simulink model "hl20airframe"  (Simulink 4.00)
settings: Solver=ode45  StartTime=0.0  StopTime=1000.0  RelTol=1e-3
PreLoadFcn:
  | init_hl20
values from neighbouring files (symbols this model uses):
  alpha_vec_Cn0 = [-10 -5 0 5 10 15 20 25 30]    [init_hl20.m]
  b_ref = 13.89/m2ft    (= 4.23367186452)    [init_hl20.m]
  beta_vec_Cn0 = [0 2 5 10]    [init_hl20.m]
  Clbeta = -0.00787    [init_hl20.m]
  Cm0 = reshape(temp(:,2),length(beta_vec_0),length(alpha_vec_0))    [init_hl20.m]
  CX0 = -reshape(temp(:,3),length(beta_vec_0),length(alpha_vec_0))    [init_hl20.m]
  CYbeta = -0.01242    [init_hl20.m]
  CZ0 = -reshape(temp(:,1),length(beta_vec_0),length(alpha_vec_0))    [init_hl20.m]
  d2r = pi/180    (= 0.0174532925199)    [init_hl20.m]
  d_ref = 28.24/m2ft    (= 8.60755172456)    [init_hl20.m]
  Inertia = diag([Ixx Iyy Izz])    [init_hl20.m]
  mass = massBody+massFuel    (= 11738.9844962)    [init_hl20.m]
  S_ref = 286.45/m2ft^2    (= 26.6120741048)    [init_hl20.m]
  x_cg = 0.575*len_veh    (= 4.78635044684)    [init_hl20.m]
  x_ref = 0.54*len_veh    (= 4.49500737616)    [init_hl20.m]
undefined symbols (not defined in the file or in its folder): Light
libraries: simulink3 x40, aerolibwind x3, aerolib6dof x1, aerolibatmos x1, aerolibgravity x1, aerolibtransform x1
settings Model: Creator=sgage  LastModifiedBy=sgage  OptimizeBlockIOStorage=off

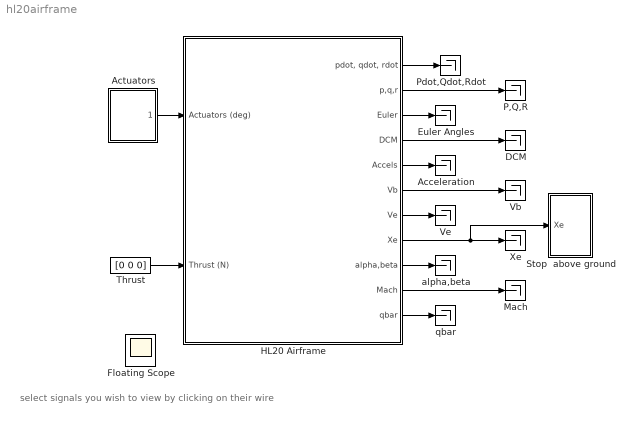
== system hl20airframe ==
  note: select signals you wish to view
      | by clicking on their wire
  Acceleration : Terminator
  Actuators : Subsystem
      settings: RTWFcnNameOpts=Auto  RTWFileNameOpts=Auto
  DCM : Terminator
  Euler Angles : Terminator
  Floating Scope : Scope
      settings: Floating=on  TimeRange=10  YMin=-7500  YMax=1000  SaveToWorkspace=off  SaveName=ScopeData  LimitDataPoints=on  MaxDataPoints=5000
  HL20 Airframe : Subsystem
      settings: RTWFcnNameOpts=Auto  RTWFileNameOpts=Auto
      mask Display: image(imread('aeroblk_HL20pic.jpg','jpg'))
  Mach : Terminator
  P,Q,R : Terminator
  Pdot,Qdot,Rdot : Terminator
  Stop  above ground : Subsystem
      settings: RTWFcnNameOpts=Auto  RTWFileNameOpts=Auto
  Thrust : Constant  Value=[0 0 0]
  Vb : Terminator
  Ve : Terminator
  Xe : Terminator
  alpha,beta : Terminator
  qbar : Terminator
  wires:
  Thrust/1 -> HL20 Airframe/2(Thrust (N))
  Actuators/1(Positions) -> HL20 Airframe/1(Actuators (deg))
  HL20 Airframe/11(qbar) -> qbar/1
  HL20 Airframe/3(Euler) -> Euler Angles/1
  HL20 Airframe/5(Accels) -> Acceleration/1
  HL20 Airframe/6(Vb) -> Vb/1
  HL20 Airframe/1("pdot, qdot, rdot") -> Pdot,Qdot,Rdot/1
  HL20 Airframe/2(p,q,r) -> P,Q,R/1
  HL20 Airframe/7(Ve) -> Ve/1
  HL20 Airframe/8(Xe) -> Xe/1, Stop  above ground/1(Xe)
  HL20 Airframe/10(Mach) -> Mach/1
  HL20 Airframe/9(alpha,beta) -> alpha,beta/1
  HL20 Airframe/4(DCM) -> DCM/1

== system hl20airframe/Actuators ==
  Bus Creator1 : BusCreator  Inputs=6
  Constant : Constant  Value=0
  Sine Wave : Sin  SineType=Time-based  Amplitude=1  Bias=10  Frequency=1  Phase=0  Samples=10  SampleTime=0  Offset=0
  "aileron " : Saturate  UpperLimit=30  LowerLimit=-30  LinearizeAsGain=on
  elevator : Saturate  UpperLimit=30  LowerLimit=-30  LinearizeAsGain=on
  flap (diff) : Saturate  UpperLimit=60  LowerLimit=-60  LinearizeAsGain=on
  flap (neg) : Saturate  UpperLimit=0  LowerLimit=-60  LinearizeAsGain=on
  flap (pos) : Saturate  UpperLimit=60  LowerLimit=0  LinearizeAsGain=on
  rudder : Saturate  UpperLimit=60  LowerLimit=-60  LinearizeAsGain=on
  Positions : Outport  Port=1
  wires:
  Bus Creator1/1 -> Positions/1
  flap (diff)/1 -> Bus Creator1/6  "Flap(diff)"
  flap (neg)/1 -> Bus Creator1/5  "Flap(neg)"
  rudder/1 -> Bus Creator1/3  "Rudder"
  elevator/1 -> Bus Creator1/2  "Elevator"
  "aileron "/1 -> Bus Creator1/1  "Aileron"
  flap (pos)/1 -> Bus Creator1/4  "Flap(pos)"
  Constant/1 -> rudder/1, flap (diff)/1, flap (neg)/1, flap (pos)/1, "aileron "/1
  Sine Wave/1 -> elevator/1

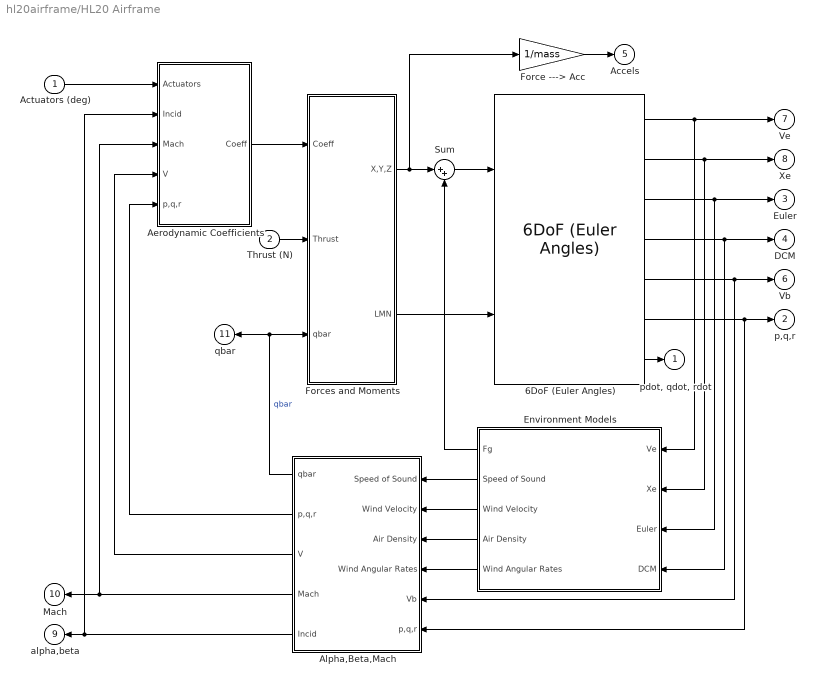
== system hl20airframe/HL20 Airframe ==
  Actuators (deg) : Inport  Port=1  LatchInput=off
  Thrust (N) : Inport  Port=2  LatchInput=off
  6DoF (Euler Angles) : aerolib6dof/6DoF (Euler Angles)  xme_0=xme_0  Vm_0=Vmw  eul_0=Euler_0  pm_0=pm_0  Mass=mass  Inertia=Inertia
  Aerodynamic Coefficients : Subsystem
      settings: RTWFcnNameOpts=Auto  RTWFileNameOpts=Auto
  Alpha,Beta,Mach : Subsystem  Orientation=left
      settings: RTWFcnNameOpts=Auto  RTWFileNameOpts=Auto
  Environment Models : Subsystem  Orientation=left
      settings: RTWFcnNameOpts=Auto  RTWFileNameOpts=Auto
  Force ---> Acc : Gain  Gain=1/mass  Multiplication=Element-wise(K.*u)  SaturateOnIntegerOverflow=on
  Forces and Moments : Subsystem
      settings: RTWFcnNameOpts=Auto  RTWFileNameOpts=Auto
  Sum : Sum  Inputs=|++  SaturateOnIntegerOverflow=on
  "pdot, qdot, rdot" : Outport  Port=1  InitialOutput=0
  p,q,r : Outport  Port=2  InitialOutput=0
  Euler : Outport  Port=3  InitialOutput=0
  DCM : Outport  Port=4  InitialOutput=0
  Accels : Outport  Port=5  InitialOutput=0
  Vb : Outport  Port=6  InitialOutput=0
  Ve : Outport  Port=7  InitialOutput=0
  Xe : Outport  Port=8  InitialOutput=0
  alpha,beta : Outport  Orientation=left  Port=9  InitialOutput=0
  Mach : Outport  Orientation=left  Port=10  InitialOutput=0
  qbar : Outport  Orientation=left  Port=11  InitialOutput=0
  wires:
  6DoF (Euler Angles)/1 -> Environment Models/1(Ve), Ve/1
  6DoF (Euler Angles)/2 -> Environment Models/2(Xe), Xe/1
  6DoF (Euler Angles)/6 -> p,q,r/1, Alpha,Beta,Mach/6(p,q,r)
  Thrust (N)/1 -> Forces and Moments/2(Thrust)
  6DoF (Euler Angles)/7 -> "pdot, qdot, rdot"/1
  6DoF (Euler Angles)/4 -> DCM/1, Environment Models/4(DCM)
  6DoF (Euler Angles)/3 -> Environment Models/3(Euler), Euler/1
  Alpha,Beta,Mach/5(Incid) -> alpha,beta/1, Aerodynamic Coefficients/2(Incid)
  Aerodynamic Coefficients/1(Coeff) -> Forces and Moments/1(Coeff)
  Environment Models/3(Wind Velocity) -> Alpha,Beta,Mach/2(Wind Velocity)
  6DoF (Euler Angles)/5 -> Alpha,Beta,Mach/5(Vb), Vb/1
  Environment Models/2(Speed of Sound) -> Alpha,Beta,Mach/1(Speed of Sound)
  Environment Models/4(Air Density) -> Alpha,Beta,Mach/3(Air Density)
  Forces and Moments/2(LMN) -> 6DoF (Euler Angles)/2
  Alpha,Beta,Mach/1(qbar) -> Forces and Moments/3(qbar), qbar/1  "qbar"
  Forces and Moments/1(X,Y,Z) -> Sum/1, Force ---> Acc/1
  Sum/1 -> 6DoF (Euler Angles)/1
  Environment Models/1(Fg) -> Sum/2
  Force ---> Acc/1 -> Accels/1
  Actuators (deg)/1 -> Aerodynamic Coefficients/1(Actuators)
  Alpha,Beta,Mach/3(V) -> Aerodynamic Coefficients/4(V)
  Alpha,Beta,Mach/4(Mach) -> Aerodynamic Coefficients/3(Mach), Mach/1
  Alpha,Beta,Mach/2("p,q,r ") -> Aerodynamic Coefficients/5(p,q,r)
  Environment Models/5(Wind Angular Rates) -> Alpha,Beta,Mach/4(Wind Angular Rates)

== system hl20airframe/Stop  above ground ==
  Xe : Inport  Port=1  LatchInput=off
  1 meter from ground : Fcn  Expr=u[1] <= 2
  Abs : Abs  SaturateOnIntegerOverflow=on
  Selector : Selector  InputType=Vector  ElementSrc=Internal  Elements=3  RowSrc=Internal  Rows=1  ColumnSrc=Internal  Columns=1  InputPortWidth=3
  Stop Simulation : Stop
  wires:
  Selector/1 -> Abs/1
  1 meter from ground/1 -> Stop Simulation/1
  Xe/1 -> Selector/1
  Abs/1 -> 1 meter from ground/1

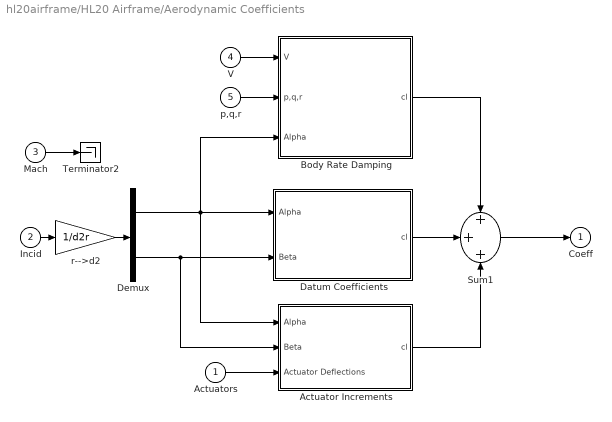
== system hl20airframe/HL20 Airframe/Aerodynamic Coefficients ==
  Actuators : Inport  Port=1  LatchInput=off
  Incid : Inport  Port=2  LatchInput=off
  Mach : Inport  Port=3  LatchInput=off
  V : Inport  Port=4  LatchInput=off
  p,q,r : Inport  Port=5  LatchInput=off
  Actuator Increments : Subsystem
      settings: RTWFcnNameOpts=Auto  RTWFileNameOpts=Auto
  Body Rate Damping : Subsystem
      settings: RTWFcnNameOpts=Auto  RTWFileNameOpts=Auto
  Datum Coefficients : Subsystem
      settings: RTWFcnNameOpts=Auto  RTWFileNameOpts=Auto
  Demux : Demux  Outputs=2  BusSelectionMode=off
  Sum1 : Sum  Inputs=+++  SaturateOnIntegerOverflow=on
  Terminator2 : Terminator
  r-->d2 : Gain  Gain=1/d2r  Multiplication=Element-wise(K.*u)  SaturateOnIntegerOverflow=on
  Coeff : Outport  Port=1  InitialOutput=0
  wires:
  Actuator Increments/1(cl) -> Sum1/3
  Body Rate Damping/1(cl) -> Sum1/1
  V/1 -> Body Rate Damping/1(V)
  Mach/1 -> Terminator2/1
  Demux/2 -> Actuator Increments/2(Beta), Datum Coefficients/2(Beta)
  Datum Coefficients/1(cl) -> Sum1/2
  Sum1/1 -> Coeff/1
  Actuators/1 -> Actuator Increments/3("Actuator Deflections ")
  r-->d2/1 -> Demux/1
  Incid/1 -> r-->d2/1
  p,q,r/1 -> Body Rate Damping/2(p,q,r)
  Demux/1 -> Actuator Increments/1(Alpha), Datum Coefficients/1(Alpha), Body Rate Damping/3(Alpha)

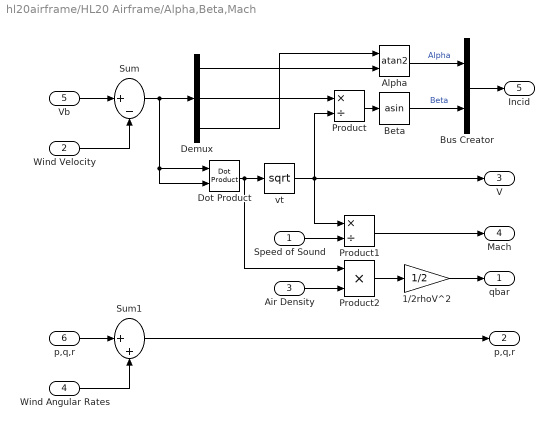
== system hl20airframe/HL20 Airframe/Alpha,Beta,Mach ==
  Speed of Sound : Inport  Port=1  LatchInput=off
  Wind Velocity : Inport  Port=2  LatchInput=off  PortDimensions=3
  Air Density : Inport  Port=3  LatchInput=off
  Wind Angular Rates : Inport  Port=4  LatchInput=off  PortDimensions=3
  Vb : Inport  Port=5  LatchInput=off  PortDimensions=3
  p,q,r : Inport  Port=6  LatchInput=off  PortDimensions=3
  1/2rhoV^2 : Gain  Gain=1/2  Multiplication=Element-wise(K.*u)  SaturateOnIntegerOverflow=on
  Alpha : Trigonometry  Operator=atan2  OutputSignalType=auto
  Beta : Trigonometry  Operator=asin  OutputSignalType=auto
  Bus Creator : BusCreator  Inputs=2
  Demux : Demux  Outputs=3  BusSelectionMode=off
  Dot Product : simulink3/Math/Dot Product
  Product : Product  Inputs=*/  Multiplication=Element-wise(.*)  SaturateOnIntegerOverflow=on
  Product1 : Product  Inputs=*/  Multiplication=Element-wise(.*)  SaturateOnIntegerOverflow=on
  Product2 : Product  Inputs=2  Multiplication=Element-wise(.*)  SaturateOnIntegerOverflow=on
  Sum : Sum  Inputs=|+-  SaturateOnIntegerOverflow=on
  Sum1 : Sum  Inputs=|++  SaturateOnIntegerOverflow=on
  vt : Math  Operator=sqrt  OutputSignalType=auto
  qbar : Outport  Port=1  InitialOutput=0
  "p,q,r " : Outport  Port=2
  V : Outport  Port=3
  Mach : Outport  Port=4
  Incid : Outport  Port=5
  wires:
  1/2rhoV^2/1 -> qbar/1
  Product2/1 -> 1/2rhoV^2/1
  Air Density/1 -> Product2/2
  Dot Product/1 -> Product2/1, vt/1
  Product1/1 -> Mach/1
  vt/1 -> V/1, Product1/1, Product/2
  Sum/1 -> Dot Product/2, Dot Product/1, Demux/1
  Vb/1 -> Sum/1
  Speed of Sound/1 -> Product1/2
  Wind Velocity/1 -> Sum/2
  Demux/2 -> Product/1
  Demux/1 -> Alpha/2
  Demux/3 -> Alpha/1
  Product/1 -> Beta/1
  Beta/1 -> Bus Creator/2  "Beta"
  Bus Creator/1 -> Incid/1
  Alpha/1 -> Bus Creator/1  "Alpha"
  p,q,r/1 -> Sum1/1
  Wind Angular Rates/1 -> Sum1/2
  Sum1/1 -> "p,q,r "/1

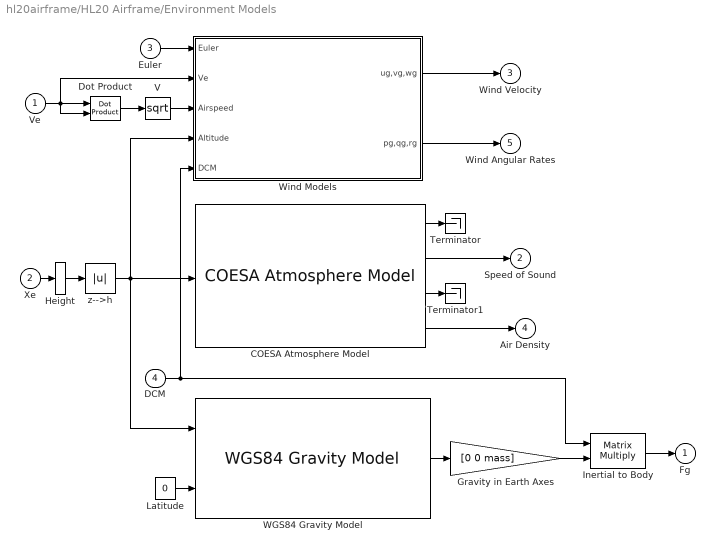
== system hl20airframe/HL20 Airframe/Environment Models ==
  Ve : Inport  Port=1  LatchInput=off
  Xe : Inport  Port=2  LatchInput=off  PortDimensions=3
  Euler : Inport  Port=3  LatchInput=off
  DCM : Inport  Port=4  LatchInput=off
  COESA Atmosphere Model : aerolibatmos/COESA Atmosphere Model  units=Metric
  Dot Product : simulink3/Math/Dot Product
  Gravity in Earth Axes : Gain  Gain=[0 0 mass]  Multiplication=Element-wise(K.*u)  SaturateOnIntegerOverflow=on
  Height : Selector  InputType=Vector  ElementSrc=Internal  Elements=[3]  RowSrc=Internal  Rows=1  ColumnSrc=Internal  Columns=1  InputPortWidth=3
  Inertial to Body : Product  Inputs=2  Multiplication=Matrix(*)  SaturateOnIntegerOverflow=on
  Latitude : Constant  Value=0
  Terminator : Terminator
  Terminator1 : Terminator
  V : Math  Operator=sqrt  OutputSignalType=auto
  WGS84 Gravity Model : aerolibgravity/WGS84 Gravity Model  model=WGS84 Taylor Series  units=Metric  no_atmos=on  precessing=on  month=February  day=1  year=2000  no_centrifugal=on
  Wind Models : Subsystem
      settings: RTWFcnNameOpts=Auto  RTWFileNameOpts=Auto
  z-->h : Abs  SaturateOnIntegerOverflow=on
  Fg : Outport  Port=1  InitialOutput=0
  Speed of Sound : Outport  Port=2  InitialOutput=0
  Wind Velocity : Outport  Port=3  InitialOutput=0
  Air Density : Outport  Port=4  InitialOutput=0
  Wind Angular Rates : Outport  Port=5  InitialOutput=0
  wires:
  Euler/1 -> Wind Models/1(Euler)
  Ve/1 -> Wind Models/2(Ve), Dot Product/1, Dot Product/2
  Wind Models/1(ug,vg,wg) -> Wind Velocity/1
  Wind Models/2(pg,qg,rg) -> Wind Angular Rates/1
  Dot Product/1 -> V/1
  z-->h/1 -> WGS84 Gravity Model/1, COESA Atmosphere Model/1, Wind Models/4(Altitude)
  COESA Atmosphere Model/4 -> Air Density/1
  COESA Atmosphere Model/2 -> Speed of Sound/1
  COESA Atmosphere Model/3 -> Terminator1/1
  COESA Atmosphere Model/1 -> Terminator/1
  Height/1 -> z-->h/1
  Xe/1 -> Height/1
  Latitude/1 -> WGS84 Gravity Model/2
  WGS84 Gravity Model/1 -> Gravity in Earth Axes/1
  Gravity in Earth Axes/1 -> Inertial to Body/2
  DCM/1 -> Wind Models/5(DCM), Inertial to Body/1
  Inertial to Body/1 -> Fg/1
  V/1 -> Wind Models/3(Airspeed)

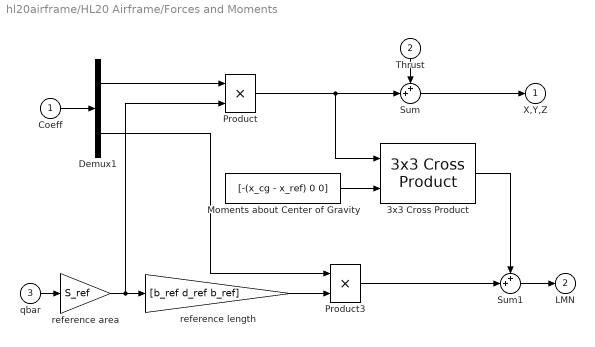
== system hl20airframe/HL20 Airframe/Forces and Moments ==
  Coeff : Inport  Port=1  LatchInput=off
  Thrust : Inport  Orientation=down  Port=2  LatchInput=off
  qbar : Inport  Port=3  LatchInput=off
  3x3 Cross Product : aerolibtransform/3x3 Cross Product
  Demux1 : Demux  Outputs=[3,3]  BusSelectionMode=off
  Moments about Center of Gravity : Constant  Value=[-(x_cg - x_ref) 0 0]
  Product : Product  Inputs=2  Multiplication=Element-wise(.*)  SaturateOnIntegerOverflow=on
  Product3 : Product  Inputs=2  Multiplication=Element-wise(.*)  SaturateOnIntegerOverflow=on
  Sum : Sum  Inputs=++|  SaturateOnIntegerOverflow=on
  Sum1 : Sum  Inputs=++|  SaturateOnIntegerOverflow=on
  reference area : Gain  Gain=S_ref  Multiplication=Element-wise(K.*u)  SaturateOnIntegerOverflow=on
  reference length : Gain  Gain=[b_ref d_ref b_ref]  Multiplication=Element-wise(K.*u)  SaturateOnIntegerOverflow=on
  X,Y,Z : Outport  Port=1  InitialOutput=0
  LMN : Outport  Port=2  InitialOutput=0
  wires:
  Sum1/1 -> LMN/1
  Product3/1 -> Sum1/2
  Moments about Center of Gravity/1 -> 3x3 Cross Product/2
  Thrust/1 -> Sum/1
  Sum/1 -> X,Y,Z/1
  reference area/1 -> reference length/1, Product/2
  qbar/1 -> reference area/1
  Demux1/2 -> Product3/1
  Demux1/1 -> Product/1
  Coeff/1 -> Demux1/1
  reference length/1 -> Product3/2
  Product/1 -> Sum/2, 3x3 Cross Product/1
  3x3 Cross Product/1 -> Sum1/1

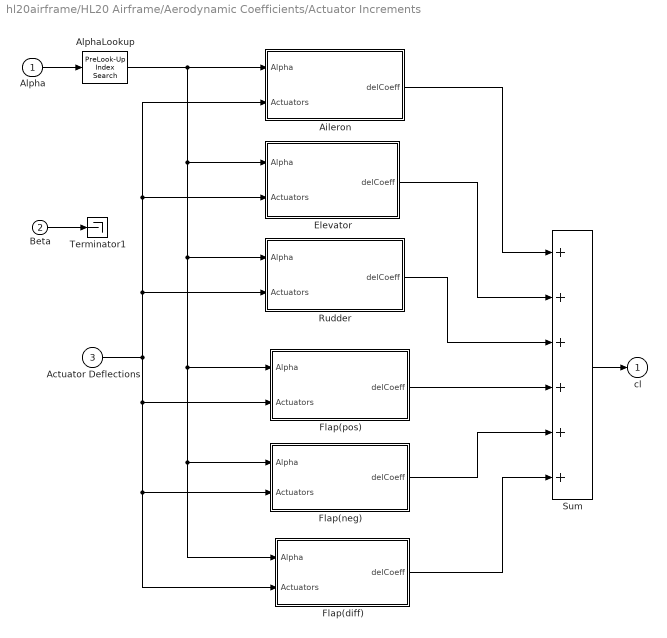
== system hl20airframe/HL20 Airframe/Aerodynamic Coefficients/Actuator Increments ==
  Alpha : Inport  Port=1  LatchInput=off
  Beta : Inport  Port=2  LatchInput=off
  "Actuator Deflections " : Inport  Port=3  LatchInput=off
  Aileron : Subsystem
      settings: RTWFcnNameOpts=Auto  RTWFileNameOpts=Auto
  AlphaLookup : simulink3/Functions & Tables/PreLook-Up Index Search  bpData=alpha_vec_0  searchMode=Binary Search  cacheBpFlag=on  outputFlag=off  extrapMode=Linear Extrapolation  rangeErrorMode=None
  Elevator : Subsystem
      settings: RTWFcnNameOpts=Auto  RTWFileNameOpts=Auto
  Flap(diff) : Subsystem
      settings: RTWFcnNameOpts=Auto  RTWFileNameOpts=Auto
  Flap(neg) : Subsystem
      settings: RTWFcnNameOpts=Auto  RTWFileNameOpts=Auto
  Flap(pos) : Subsystem
      settings: RTWFcnNameOpts=Auto  RTWFileNameOpts=Auto
  Rudder : Subsystem
      settings: RTWFcnNameOpts=Auto  RTWFileNameOpts=Auto
  Sum : Sum  Inputs=++++++  SaturateOnIntegerOverflow=on
  Terminator1 : Terminator
  cl : Outport  Port=1  InitialOutput=0
  wires:
  AlphaLookup/1 -> Elevator/1(Alpha), Rudder/1(Alpha), Flap(pos)/1(Alpha), Flap(diff)/1(Alpha), Flap(neg)/1(Alpha), Aileron/1(Alpha)
  Sum/1 -> cl/1
  Flap(diff)/1(delCoeff) -> Sum/6
  Flap(neg)/1(delCoeff) -> Sum/5
  Flap(pos)/1(delCoeff) -> Sum/4
  Rudder/1(delCoeff) -> Sum/3
  Elevator/1(delCoeff) -> Sum/2
  Aileron/1(delCoeff) -> Sum/1
  Beta/1 -> Terminator1/1
  Alpha/1 -> AlphaLookup/1
  "Actuator Deflections "/1 -> Flap(diff)/2(Actuators), Flap(neg)/2(Actuators), Flap(pos)/2(Actuators), Rudder/2(Actuators), Elevator/2(Actuators), Aileron/2(Actuators)

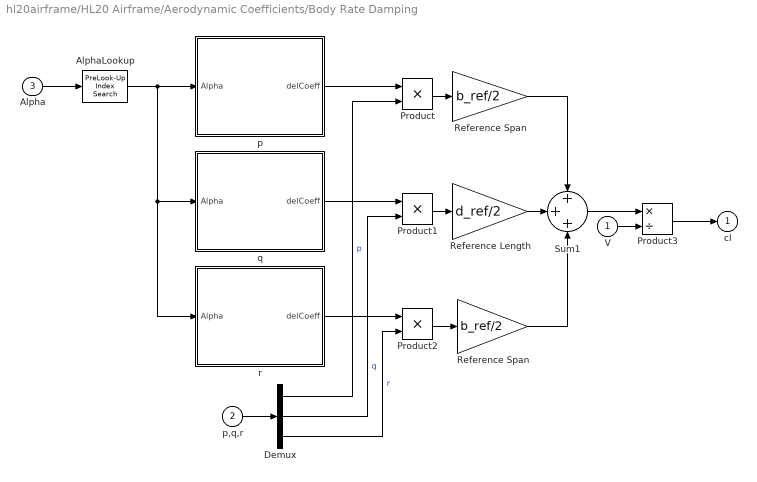
== system hl20airframe/HL20 Airframe/Aerodynamic Coefficients/Body Rate Damping ==
  V : Inport  Port=1  LatchInput=off
  p,q,r : Inport  Port=2  LatchInput=off
  Alpha : Inport  Port=3  LatchInput=off
  AlphaLookup : simulink3/Functions & Tables/PreLook-Up Index Search  bpData=alpha_vec_damping  searchMode=Binary Search  cacheBpFlag=on  outputFlag=off  extrapMode=Linear Extrapolation  rangeErrorMode=None
  Demux : Demux  Outputs=3  BusSelectionMode=off
  Product : Product  Inputs=2  Multiplication=Element-wise(.*)  SaturateOnIntegerOverflow=on
  Product1 : Product  Inputs=2  Multiplication=Element-wise(.*)  SaturateOnIntegerOverflow=on
  Product2 : Product  Inputs=2  Multiplication=Element-wise(.*)  SaturateOnIntegerOverflow=on
  Product3 : Product  Inputs=*/  Multiplication=Element-wise(.*)  SaturateOnIntegerOverflow=on
  Reference Length : Gain  Gain=d_ref/2  Multiplication=Element-wise(K.*u)  SaturateOnIntegerOverflow=on
  Reference Span : Gain  Gain=b_ref/2  Multiplication=Element-wise(K.*u)  SaturateOnIntegerOverflow=on
  "Reference Span " : Gain  Gain=b_ref/2  Multiplication=Element-wise(K.*u)  SaturateOnIntegerOverflow=on
  Sum1 : Sum  Inputs=+++  SaturateOnIntegerOverflow=on
  p : Subsystem
      settings: RTWFcnNameOpts=Auto  RTWFileNameOpts=Auto
  q : Subsystem
      settings: RTWFcnNameOpts=Auto  RTWFileNameOpts=Auto
  r : Subsystem
      settings: RTWFcnNameOpts=Auto  RTWFileNameOpts=Auto
  cl : Outport  Port=1  InitialOutput=0
  wires:
  "Reference Span "/1 -> Sum1/3
  Reference Span/1 -> Sum1/1
  Reference Length/1 -> Sum1/2
  AlphaLookup/1 -> p/1(Alpha), q/1(Alpha), r/1(Alpha)
  r/1(delCoeff) -> Product2/1
  Product/1 -> Reference Span/1
  Product2/1 -> "Reference Span "/1
  Product1/1 -> Reference Length/1
  Product3/1 -> cl/1
  V/1 -> Product3/2
  Sum1/1 -> Product3/1
  Demux/3 -> Product2/2  "r"
  Demux/2 -> Product1/2  "q"
  Demux/1 -> Product/2  "p"
  p,q,r/1 -> Demux/1
  q/1(delCoeff) -> Product1/1
  p/1(delCoeff) -> Product/1
  Alpha/1 -> AlphaLookup/1

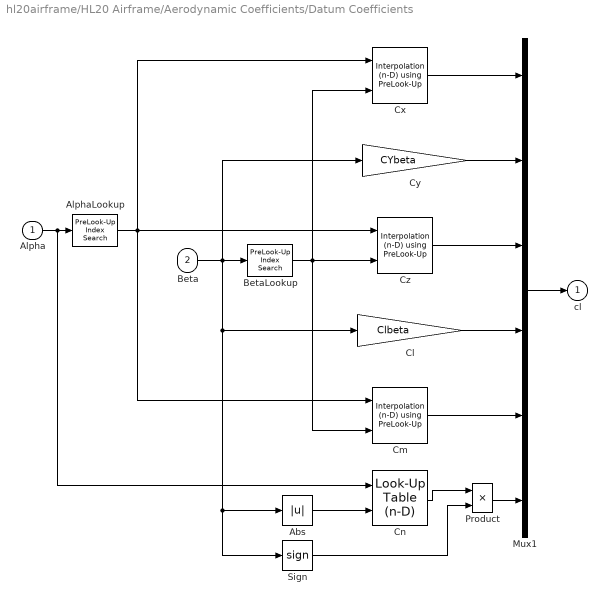
== system hl20airframe/HL20 Airframe/Aerodynamic Coefficients/Datum Coefficients ==
  Alpha : Inport  Port=1  LatchInput=off
  Beta : Inport  Port=2  LatchInput=off
  " Cn" : simulink3/Functions & Tables/Look-Up Table (n-D)  numDimsPopupSelect=2  bp1=alpha_vec_Cn0  bp2=beta_vec_Cn0  bp3=[1:3]  bp4=[1:3]  bpcell={ [1:3], [1:3] }  explicitNumDims=2  searchMode=Binary Search  cacheBpFlag=off  vectorInputFlag=off  tableData=Cn0  interpMethod=Linear  extrapMethod=Linear  rangeErrorMode=None
  Abs : Abs  SaturateOnIntegerOverflow=on
  AlphaLookup : simulink3/Functions & Tables/PreLook-Up Index Search  bpData=alpha_vec_0  searchMode=Binary Search  cacheBpFlag=on  outputFlag=off  extrapMode=Linear Extrapolation  rangeErrorMode=None
  BetaLookup : simulink3/Functions & Tables/PreLook-Up Index Search  bpData=beta_vec_0  searchMode=Binary Search  cacheBpFlag=on  outputFlag=off  extrapMode=Linear Extrapolation  rangeErrorMode=None
  Cl : Gain  Gain=Clbeta  Multiplication=Element-wise(K.*u)  SaturateOnIntegerOverflow=on
  Cm : simulink3/Functions & Tables/Interpolation (n-D) using PreLook-Up  numDimsPopupSelect=2  explicitNumDims=2  table=Cm0'  interpMethod=Linear  extrapMethod=Linear  rangeErrorMode=None
  Cx : simulink3/Functions & Tables/Interpolation (n-D) using PreLook-Up  numDimsPopupSelect=2  explicitNumDims=2  table=CX0'  interpMethod=Linear  extrapMethod=Linear  rangeErrorMode=None
  Cy : Gain  Gain=CYbeta  Multiplication=Element-wise(K.*u)  SaturateOnIntegerOverflow=on
  Cz : simulink3/Functions & Tables/Interpolation (n-D) using PreLook-Up  numDimsPopupSelect=2  explicitNumDims=2  table=CZ0'  interpMethod=Linear  extrapMethod=Linear  rangeErrorMode=None
  Mux1 : Mux  Inputs=6
      settings: DisplayOption=none
  Product : Product  Inputs=2  Multiplication=Element-wise(.*)  SaturateOnIntegerOverflow=on
  Sign : Signum
  cl : Outport  Port=1  InitialOutput=0
  wires:
  BetaLookup/1 -> Cx/2, Cm/2, Cz/2
  AlphaLookup/1 -> Cz/1, Cm/1, Cx/1
  Beta/1 -> Cl/1, Abs/1, Sign/1, Cy/1, BetaLookup/1
  Alpha/1 -> " Cn"/1, AlphaLookup/1
  Cl/1 -> Mux1/4
  Cy/1 -> Mux1/2
  Cm/1 -> Mux1/5
  Cz/1 -> Mux1/3
  Cx/1 -> Mux1/1
  Mux1/1 -> cl/1
  Abs/1 -> " Cn"/2
  Product/1 -> Mux1/6
  " Cn"/1 -> Product/1
  Sign/1 -> Product/2

== system hl20airframe/HL20 Airframe/Environment Models/Wind Models ==
  Euler : Inport  Port=1  LatchInput=off
  Ve : Inport  Port=2  LatchInput=off
  Airspeed : Inport  Port=3  LatchInput=off
  Altitude : Inport  Port=4  LatchInput=off
  DCM : Inport  Port=5  LatchInput=off
  Discrete Wind Gust Model - On : aerolibwind/Discrete Wind Gust Model  v_units=meters/second  Gx=on  Gy=on  Gz=on  t_0=20  d_m=[120 120 80]  v_m=[3.5 3.0 3.0]
  Dryden Wind Turbulence Model : aerolibwind/Dryden Wind Turbulence Model  v_units=meters/second  W20=5  TurbProb=10^-2 - Light  L_high=533  Wingspan=4  ts=0.1  Seed=[23341 23342 23343 23344]  T_on=on
  Sum : Sum  Inputs=+++  SaturateOnIntegerOverflow=on
  Terminator : Terminator
  Terminator1 : Terminator
  Wind Shear Model : aerolibwind/Wind Shear Model  v_units=meters/second  phase=Category C - Terminal Flight Phase  W_20=1  Wdeg=0
  ug,vg,wg : Outport  Port=1
  pg,qg,rg : Outport  Port=2
  wires:
  Euler/1 -> Terminator1/1
  Ve/1 -> Terminator/1
  Wind Shear Model/1 -> Sum/1
  Dryden Wind Turbulence Model/1 -> Sum/2
  Discrete Wind Gust Model - On/1 -> Sum/3
  Sum/1 -> ug,vg,wg/1
  DCM/1 -> Wind Shear Model/2
  Airspeed/1 -> Discrete Wind Gust Model - On/1, Dryden Wind Turbulence Model/2
  Dryden Wind Turbulence Model/2 -> pg,qg,rg/1
  Altitude/1 -> Wind Shear Model/1, Dryden Wind Turbulence Model/1

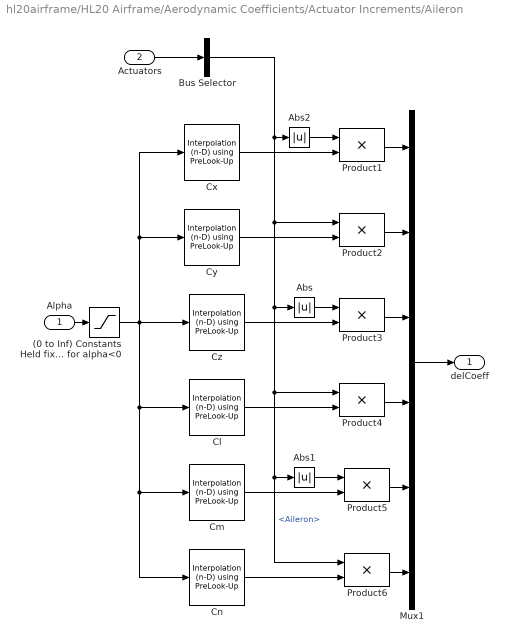
== system hl20airframe/HL20 Airframe/Aerodynamic Coefficients/Actuator Increments/Aileron ==
  Alpha : Inport  Port=1  LatchInput=off
  Actuators : Inport  Port=2  LatchInput=off
  (0 to Inf) Constants Held fixed for alpha<0 : Saturate  UpperLimit=Inf  LowerLimit=0  LinearizeAsGain=on
  Abs : Abs  SaturateOnIntegerOverflow=on
  Abs1 : Abs  SaturateOnIntegerOverflow=on
  Abs2 : Abs  SaturateOnIntegerOverflow=on
  Bus Selector : BusSelector  OutputSignals=Aileron  MuxedOutput=off
  Cl : simulink3/Functions & Tables/Interpolation (n-D) using PreLook-Up  numDimsPopupSelect=1  explicitNumDims=2  table=Clda  interpMethod=Linear  extrapMethod=Linear  rangeErrorMode=None
  Cm : simulink3/Functions & Tables/Interpolation (n-D) using PreLook-Up  numDimsPopupSelect=1  explicitNumDims=2  table=Cmda  interpMethod=Linear  extrapMethod=Linear  rangeErrorMode=None
  Cn : simulink3/Functions & Tables/Interpolation (n-D) using PreLook-Up  numDimsPopupSelect=1  explicitNumDims=2  table=Cnda  interpMethod=Linear  extrapMethod=Linear  rangeErrorMode=None
  Cx : simulink3/Functions & Tables/Interpolation (n-D) using PreLook-Up  numDimsPopupSelect=1  explicitNumDims=2  table=CXda  interpMethod=Linear  extrapMethod=Linear  rangeErrorMode=None
  Cy : simulink3/Functions & Tables/Interpolation (n-D) using PreLook-Up  numDimsPopupSelect=1  explicitNumDims=2  table=CYda  interpMethod=Linear  extrapMethod=Linear  rangeErrorMode=None
  Cz : simulink3/Functions & Tables/Interpolation (n-D) using PreLook-Up  numDimsPopupSelect=1  explicitNumDims=2  table=CZda  interpMethod=Linear  extrapMethod=Linear  rangeErrorMode=None
  Mux1 : Mux  Inputs=6
      settings: DisplayOption=none
  Product{1..6} (6 alike) : Product  Inputs=2  Multiplication=Element-wise(.*)  SaturateOnIntegerOverflow=on
  delCoeff : Outport  Port=1
  wires:
  (0 to Inf) Constants Held fixed for alpha<0/1 -> Cn/1, Cm/1, Cl/1, Cz/1, Cy/1, Cx/1
  Abs2/1 -> Product1/1
  Abs1/1 -> Product5/1
  Abs/1 -> Product3/1
  Bus Selector/1 -> Abs2/1, Product2/1, Abs/1, Product4/1, Abs1/1, Product6/1  "<Aileron>"
  Product6/1 -> Mux1/6
  Cn/1 -> Product6/2
  Product5/1 -> Mux1/5
  Cm/1 -> Product5/2
  Product4/1 -> Mux1/4
  Cl/1 -> Product4/2
  Cz/1 -> Product3/2
  Product3/1 -> Mux1/3
  Cy/1 -> Product2/2
  Product2/1 -> Mux1/2
  Cx/1 -> Product1/2
  Product1/1 -> Mux1/1
  Mux1/1 -> delCoeff/1
  Actuators/1 -> Bus Selector/1
  Alpha/1 -> (0 to Inf) Constants Held fixed for alpha<0/1

== system hl20airframe/HL20 Airframe/Aerodynamic Coefficients/Actuator Increments/Elevator ==
  Alpha : Inport  Port=1  LatchInput=off
  Actuators : Inport  Port=2  LatchInput=off
  Bus Selector1 : BusSelector  OutputSignals=Elevator  MuxedOutput=off
  Cm : simulink3/Functions & Tables/Interpolation (n-D) using PreLook-Up  numDimsPopupSelect=1  explicitNumDims=2  table=Cmde  interpMethod=Linear  extrapMethod=Linear  rangeErrorMode=None
  Constant1 : Constant  Value=0
  Cx : simulink3/Functions & Tables/Interpolation (n-D) using PreLook-Up  numDimsPopupSelect=1  explicitNumDims=2  table=CXde  interpMethod=Linear  extrapMethod=Linear  rangeErrorMode=None
  Cz : simulink3/Functions & Tables/Interpolation (n-D) using PreLook-Up  numDimsPopupSelect=1  explicitNumDims=2  table=CZde  interpMethod=Linear  extrapMethod=Linear  rangeErrorMode=None
  Mux1 : Mux  Inputs=6
      settings: DisplayOption=none
  Product : Product  Inputs=2  Multiplication=Element-wise(.*)  SaturateOnIntegerOverflow=on
  delCoeff : Outport  Port=1
  wires:
  Bus Selector1/1 -> Product/2  "<Elevator>"
  Actuators/1 -> Bus Selector1/1
  Constant1/1 -> Mux1/6, Mux1/4, Mux1/2
  Cm/1 -> Mux1/5
  Cz/1 -> Mux1/3
  Cx/1 -> Mux1/1
  Alpha/1 -> Cm/1, Cx/1, Cz/1
  Mux1/1 -> Product/1
  Product/1 -> delCoeff/1

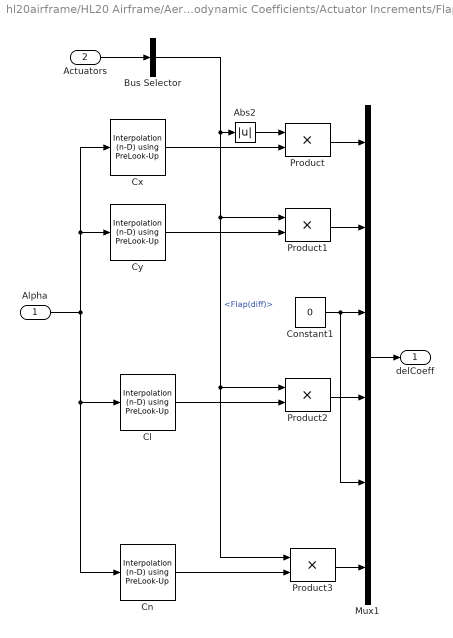
== system hl20airframe/HL20 Airframe/Aerodynamic Coefficients/Actuator Increments/Flap(diff) ==
  Alpha : Inport  Port=1  LatchInput=off
  Actuators : Inport  Port=2  LatchInput=off
  Abs2 : Abs  SaturateOnIntegerOverflow=on
  Bus Selector : BusSelector  OutputSignals=Flap(diff)  MuxedOutput=off
  Cl : simulink3/Functions & Tables/Interpolation (n-D) using PreLook-Up  numDimsPopupSelect=1  explicitNumDims=2  table=Clddf  interpMethod=Linear  extrapMethod=Linear  rangeErrorMode=None
  Cn : simulink3/Functions & Tables/Interpolation (n-D) using PreLook-Up  numDimsPopupSelect=1  explicitNumDims=2  table=Cnddf  interpMethod=Linear  extrapMethod=Linear  rangeErrorMode=None
  Constant1 : Constant  Value=0
  Cx : simulink3/Functions & Tables/Interpolation (n-D) using PreLook-Up  numDimsPopupSelect=1  explicitNumDims=2  table=CXddf  interpMethod=Linear  extrapMethod=Linear  rangeErrorMode=None
  Cy : simulink3/Functions & Tables/Interpolation (n-D) using PreLook-Up  numDimsPopupSelect=1  explicitNumDims=2  table=CYddf  interpMethod=Linear  extrapMethod=Linear  rangeErrorMode=None
  Mux1 : Mux  Inputs=6
      settings: DisplayOption=none
  Product{,1..3} (4 alike) : Product  Inputs=2  Multiplication=Element-wise(.*)  SaturateOnIntegerOverflow=on
  delCoeff : Outport  Port=1
  wires:
  Constant1/1 -> Mux1/5, Mux1/3
  Abs2/1 -> Product/1
  Cn/1 -> Product3/2
  Product3/1 -> Mux1/6
  Cy/1 -> Product1/2
  Cl/1 -> Product2/2
  Product2/1 -> Mux1/4
  Product1/1 -> Mux1/2
  Bus Selector/1 -> Abs2/1, Product1/1, Product2/1, Product3/1  "<Flap(diff)>"
  Cx/1 -> Product/2
  Product/1 -> Mux1/1
  Actuators/1 -> Bus Selector/1
  Alpha/1 -> Cx/1, Cy/1, Cn/1, Cl/1
  Mux1/1 -> delCoeff/1

== system hl20airframe/HL20 Airframe/Aerodynamic Coefficients/Actuator Increments/Flap(neg) ==
  Alpha : Inport  Port=1  LatchInput=off
  Actuators : Inport  Port=2  LatchInput=off
  Bus Selector : BusSelector  OutputSignals=Flap(neg)  MuxedOutput=off
  Cm : simulink3/Functions & Tables/Interpolation (n-D) using PreLook-Up  numDimsPopupSelect=1  explicitNumDims=2  table=Cmdfn  interpMethod=Linear  extrapMethod=Linear  rangeErrorMode=None
  Constant1 : Constant  Value=0
  Constant2 : Constant  Value=0
  Constant3 : Constant  Value=0
  Cx : simulink3/Functions & Tables/Interpolation (n-D) using PreLook-Up  numDimsPopupSelect=1  explicitNumDims=2  table=CXdfn  interpMethod=Linear  extrapMethod=Linear  rangeErrorMode=None
  Cz : simulink3/Functions & Tables/Interpolation (n-D) using PreLook-Up  numDimsPopupSelect=1  explicitNumDims=2  table=CZdfn  interpMethod=Linear  extrapMethod=Linear  rangeErrorMode=None
  Mux1 : Mux  Inputs=6
      settings: DisplayOption=none
  Product : Product  Inputs=2  Multiplication=Element-wise(.*)  SaturateOnIntegerOverflow=on
  delCoeff : Outport  Port=1
  wires:
  Bus Selector/1 -> Product/2  "<Flap(neg)>"
  Constant3/1 -> Mux1/6
  Constant2/1 -> Mux1/4
  Constant1/1 -> Mux1/2
  Actuators/1 -> Bus Selector/1
  Product/1 -> delCoeff/1
  Mux1/1 -> Product/1
  Alpha/1 -> Cx/1, Cm/1, Cz/1
  Cx/1 -> Mux1/1
  Cz/1 -> Mux1/3
  Cm/1 -> Mux1/5

== system hl20airframe/HL20 Airframe/Aerodynamic Coefficients/Actuator Increments/Flap(pos) ==
  Alpha : Inport  Port=1  LatchInput=off
  Actuators : Inport  Port=2  LatchInput=off
  Bus Selector : BusSelector  OutputSignals=Flap(pos)  MuxedOutput=off
  Cm : simulink3/Functions & Tables/Interpolation (n-D) using PreLook-Up  numDimsPopupSelect=1  explicitNumDims=2  table=Cmdfp  interpMethod=Linear  extrapMethod=Linear  rangeErrorMode=None
  Constant1 : Constant  Value=0
  Constant2 : Constant  Value=0
  Constant3 : Constant  Value=0
  Cx : simulink3/Functions & Tables/Interpolation (n-D) using PreLook-Up  numDimsPopupSelect=1  explicitNumDims=2  table=CXdfp  interpMethod=Linear  extrapMethod=Linear  rangeErrorMode=None
  Cz : simulink3/Functions & Tables/Interpolation (n-D) using PreLook-Up  numDimsPopupSelect=1  explicitNumDims=2  table=CZdfp  interpMethod=Linear  extrapMethod=Linear  rangeErrorMode=None
  Mux1 : Mux  Inputs=6
      settings: DisplayOption=none
  Product : Product  Inputs=2  Multiplication=Element-wise(.*)  SaturateOnIntegerOverflow=on
  delCoeff : Outport  Port=1
  wires:
  Bus Selector/1 -> Product/2  "<Flap(pos)>"
  Actuators/1 -> Bus Selector/1
  Constant3/1 -> Mux1/6
  Constant2/1 -> Mux1/4
  Constant1/1 -> Mux1/2
  Cm/1 -> Mux1/5
  Cz/1 -> Mux1/3
  Cx/1 -> Mux1/1
  Alpha/1 -> Cx/1, Cm/1, Cz/1
  Mux1/1 -> Product/1
  Product/1 -> delCoeff/1

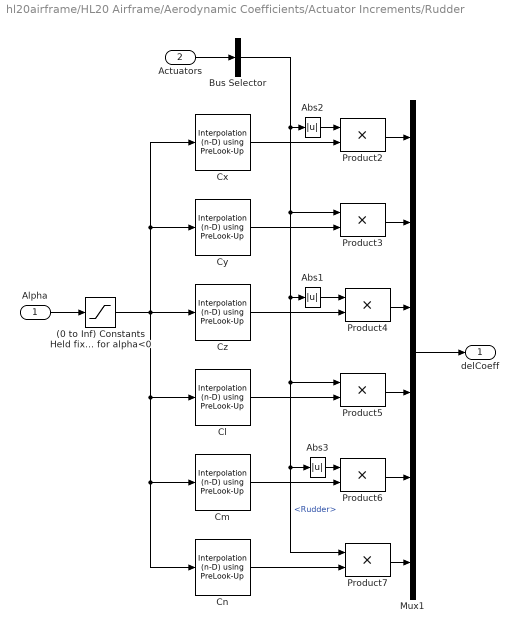
== system hl20airframe/HL20 Airframe/Aerodynamic Coefficients/Actuator Increments/Rudder ==
  Alpha : Inport  Port=1  LatchInput=off
  Actuators : Inport  Port=2  LatchInput=off
  (0 to Inf) Constants Held fixed for alpha<0 : Saturate  UpperLimit=Inf  LowerLimit=0  LinearizeAsGain=on
  Abs1 : Abs  SaturateOnIntegerOverflow=on
  Abs2 : Abs  SaturateOnIntegerOverflow=on
  Abs3 : Abs  SaturateOnIntegerOverflow=on
  Bus Selector : BusSelector  OutputSignals=Rudder  MuxedOutput=off
  Cl : simulink3/Functions & Tables/Interpolation (n-D) using PreLook-Up  numDimsPopupSelect=1  explicitNumDims=2  table=Cldr  interpMethod=Linear  extrapMethod=Linear  rangeErrorMode=None
  Cm : simulink3/Functions & Tables/Interpolation (n-D) using PreLook-Up  numDimsPopupSelect=1  explicitNumDims=2  table=Cmdr  interpMethod=Linear  extrapMethod=Linear  rangeErrorMode=None
  Cn : simulink3/Functions & Tables/Interpolation (n-D) using PreLook-Up  numDimsPopupSelect=1  explicitNumDims=2  table=Cndr  interpMethod=Linear  extrapMethod=Linear  rangeErrorMode=None
  Cx : simulink3/Functions & Tables/Interpolation (n-D) using PreLook-Up  numDimsPopupSelect=1  explicitNumDims=2  table=CXdr  interpMethod=Linear  extrapMethod=Linear  rangeErrorMode=None
  Cy : simulink3/Functions & Tables/Interpolation (n-D) using PreLook-Up  numDimsPopupSelect=1  explicitNumDims=2  table=CYdr  interpMethod=Linear  extrapMethod=Linear  rangeErrorMode=None
  Cz : simulink3/Functions & Tables/Interpolation (n-D) using PreLook-Up  numDimsPopupSelect=1  explicitNumDims=2  table=CZdr  interpMethod=Linear  extrapMethod=Linear  rangeErrorMode=None
  Mux1 : Mux  Inputs=6
      settings: DisplayOption=none
  Product{2..7} (6 alike) : Product  Inputs=2  Multiplication=Element-wise(.*)  SaturateOnIntegerOverflow=on
  delCoeff : Outport  Port=1
  wires:
  Abs3/1 -> Product6/1
  Abs1/1 -> Product4/1
  Abs2/1 -> Product2/1
  Bus Selector/1 -> Abs2/1, Abs1/1, Abs3/1, Product7/1, Product5/1, Product3/1  "<Rudder>"
  Product7/1 -> Mux1/6
  Cn/1 -> Product7/2
  Product6/1 -> Mux1/5
  Cm/1 -> Product6/2
  Product5/1 -> Mux1/4
  Cl/1 -> Product5/2
  Product4/1 -> Mux1/3
  Cz/1 -> Product4/2
  Product3/1 -> Mux1/2
  Cy/1 -> Product3/2
  Product2/1 -> Mux1/1
  Cx/1 -> Product2/2
  Actuators/1 -> Bus Selector/1
  Mux1/1 -> delCoeff/1
  Alpha/1 -> (0 to Inf) Constants Held fixed for alpha<0/1
  (0 to Inf) Constants Held fixed for alpha<0/1 -> Cn/1, Cm/1, Cl/1, Cz/1, Cy/1, Cx/1

== system hl20airframe/HL20 Airframe/Aerodynamic Coefficients/Body Rate Damping/p ==
  Alpha : Inport  Port=1  LatchInput=off
  Cl : simulink3/Functions & Tables/Interpolation (n-D) using PreLook-Up  numDimsPopupSelect=1  explicitNumDims=2  table=Clp  interpMethod=Linear  extrapMethod=Linear  rangeErrorMode=None
  Cn : simulink3/Functions & Tables/Interpolation (n-D) using PreLook-Up  numDimsPopupSelect=1  explicitNumDims=2  table=Cnp  interpMethod=Linear  extrapMethod=Linear  rangeErrorMode=None
  Constant1 : Constant  Value=0
  Mux1 : Mux  Inputs=6
      settings: DisplayOption=none
  delCoeff : Outport  Port=1
  wires:
  Alpha/1 -> Cn/1, Cl/1
  Cl/1 -> Mux1/4  "Cl"
  Cn/1 -> Mux1/6
  Constant1/1 -> Mux1/2, Mux1/3, Mux1/5, Mux1/1  "Cxp"
  Mux1/1 -> delCoeff/1

== system hl20airframe/HL20 Airframe/Aerodynamic Coefficients/Body Rate Damping/q ==
  Alpha : Inport  Port=1  LatchInput=off
  Cmq : simulink3/Functions & Tables/Interpolation (n-D) using PreLook-Up  numDimsPopupSelect=1  explicitNumDims=2  table=Cmq  interpMethod=Linear  extrapMethod=Linear  rangeErrorMode=None
  Constant3 : Constant  Value=0
  Mux1 : Mux  Inputs=6
      settings: DisplayOption=none
  delCoeff : Outport  Port=1
  wires:
  Alpha/1 -> Cmq/1
  Mux1/1 -> delCoeff/1
  Constant3/1 -> Mux1/4, Mux1/6, Mux1/3, Mux1/2, Mux1/1
  Cmq/1 -> Mux1/5

== system hl20airframe/HL20 Airframe/Aerodynamic Coefficients/Body Rate Damping/r ==
  Alpha : Inport  Port=1  LatchInput=off
  Clr : simulink3/Functions & Tables/Interpolation (n-D) using PreLook-Up  numDimsPopupSelect=1  explicitNumDims=2  table=Clr  interpMethod=Linear  extrapMethod=Linear  rangeErrorMode=None
  Cnr : simulink3/Functions & Tables/Interpolation (n-D) using PreLook-Up  numDimsPopupSelect=1  explicitNumDims=2  table=Cnr  interpMethod=Linear  extrapMethod=Linear  rangeErrorMode=None
  Constant : Constant  Value=0
  Mux1 : Mux  Inputs=6
      settings: DisplayOption=none
  delCoeff : Outport  Port=1
  wires:
  Alpha/1 -> Cnr/1, Clr/1
  Mux1/1 -> delCoeff/1
  Constant/1 -> Mux1/3, Mux1/5, Mux1/2, Mux1/1  "Cxr"
  Clr/1 -> Mux1/4  "Cl"
  Cnr/1 -> Mux1/6
